simulink model "funcionModelo1"  (R2024b)
settings: Solver=VariableStepAuto  StartTime=0.0  StopTime=10.0  RelTol=1e-3
settings Model: Creator=tomi  LastModifiedBy=tomi

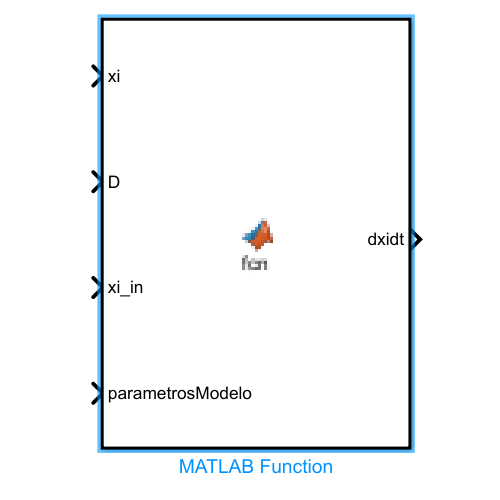
[thumbnail: Simulink's stored preview of the top-level diagram]
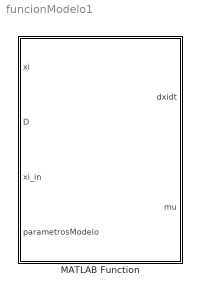
== system funcionModelo1 ==
  MATLAB Function : MATLAB Function  TreatAsAtomicUnit=on

== matlab function funcionModelo1/MATLAB Function ==
  data: xi input; dxidt output; D input; xi_in input; parametrosModelo input; mu output
function [dxidt, mu] = fcn(xi, D, xi_in, parametrosModelo)

    x=xi(1);
    s=xi(2);

    mux_max=parametrosModelo.mux_max;
    Ks = parametrosModelo.Ks;
    K = parametrosModelo.k;

    mu = mu_max*s/(s+Ks);
    r = mu*x;

dxidt
